simulink model "punto3"  (R2015a)
settings: Solver=ode45  StartTime=0.0  StopTime=10.0  RelTol=1e-3
libraries: cstblocks x2
settings Model: Creator=Jose Roldan  LastModifiedBy=Jose Roldan

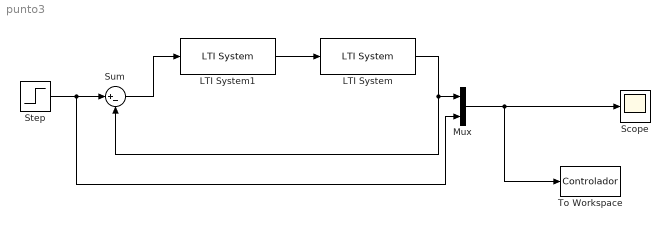
== system punto3 ==
  LTI System : cstblocks/LTI System  sys=G  IC=[]
  LTI System1 : cstblocks/LTI System  sys=C  IC=[]
  Mux : Mux  Inputs=2
  Scope : Scope
  Step : Step  SampleTime=0
  Sum : Sum  Inputs=|+-
  To Workspace : ToWorkspace  VariableName=Controlador  SaveFormat=Timeseries  SampleTime=-1
  wires:
  LTI System/1 -> Mux/1, Sum/2
  Mux/1 -> To Workspace/1, Scope/1
  LTI System1/1 -> LTI System/1
  Step/1 -> Mux/2, Sum/1
  Sum/1 -> LTI System1/1
